simulink model "lqr_period_ideal"  (R2015a)
settings: Solver=ode45  SolverMode=SingleTasking  StartTime=0.0  StopTime=simu.time  RelTol=1e-3
values from neighbouring files (symbols this model uses):
  g_Ts = i / 1000    [lqr_period_ideal_m.m]    (also in lqr_period_with_abitary_reference.m = 100)
  plant = tf([10],[tau -1])    [lqr_period_ideal_m.m]    (also in lqr_period_with_abitary_reference.m = tf([10],[tau 1]))
undefined symbols (not defined in the file or in its folder): simu
settings Model: CovSFcnEnable=off  ExtModeTrigMode=oneshot  ExtModeArmWhenConnect=off  Creator=The MathWorks Inc.  LastModifiedBy=Xiaotian
settings DataIOCC: LimitDataPoints=off  SaveOutput=off  SignalLogging=off  DSMLogging=off  SaveTime=off  SignalLoggingName=sigsOut
settings OptimizationCC: BooleanDataType=off  ExpressionDepthLimit=2147483647  InitFltsAndDblsToZero=on
settings DebuggingCC: SaveWithParameterizedLinksMsg=none  UnderspecifiedInitializationDetection=Classic  MergeDetectMultiDrivingBlocksExec=none  SignalResolutionControl=TryResolveAllWithWarning  MultiTaskDSMMsg=warning  MultiTaskCondExecSysMsg=none  IntegerOverflowMsg=none  FcnCallInpInsideContextMsg=UseLocalSettings  StateNameClashWarn=warning  IntegerSaturationMsg=none
settings HardwareCC: TargetUnknown=on
settings GRTTargetCC: TargetFcnLib=ansi_tfl_tmw.mat  CombineOutputUpdateFcns=off  GRTInterface=on

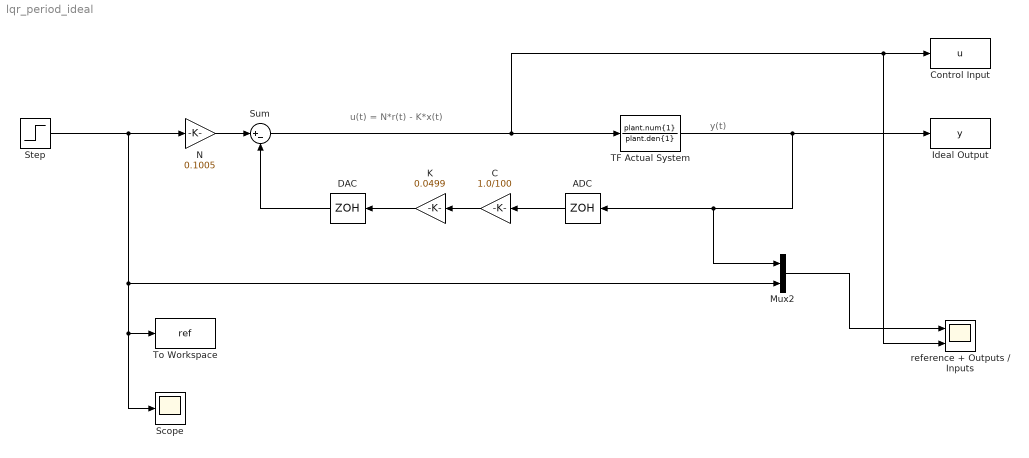
== system lqr_period_ideal ==
  note: u(t) = N*r(t) - K*x(t)
  note: y(t)
  ADC : ZeroOrderHold  SampleTime=g_Ts
  C : Gain  Gain=1.0/100
  Control Input : ToWorkspace  VariableName=u  SampleTime=simu.samlping_time
      settings: MaxDataPoints=Inf
  DAC : ZeroOrderHold  SampleTime=g_Ts
  Ideal Output : ToWorkspace  VariableName=y  SampleTime=simu.samlping_time
      settings: MaxDataPoints=Inf
  K : Gain  Gain=0.0499
  Mux2 : Mux  Inputs=2
  N : Gain  Gain=0.1005
  Scope : Scope
      settings: YMin=0.95  YMax=1.05  SaveName=ScopeData7
  Step : Step  Time=0.1  SampleTime=0
  Sum : Sum  Inputs=|+-
  TF Actual System : TransferFcn  Numerator=plant.num{1}  Denominator=plant.den{1}
  To Workspace : ToWorkspace  VariableName=ref  SampleTime=simu.samlping_time
  reference + Outputs / Inputs : Scope  NumInputPorts=2
      settings: TimeRange=1  YMin=-0.25~-600  YMax=3~200  DataFormat=Structure  SampleInput=on  SampleTime=simu.samlping_time
  wires:
  TF Actual System/1 -> Ideal Output/1, Mux2/1, ADC/1
  Sum/1 -> reference + Outputs / Inputs/2, Control Input/1, TF Actual System/1
  Mux2/1 -> reference + Outputs / Inputs/1
  Step/1 -> N/1, Mux2/2, Scope/1, To Workspace/1
  N/1 -> Sum/1
  K/1 -> DAC/1
  DAC/1 -> Sum/2
  C/1 -> K/1
  ADC/1 -> C/1
